simulink model "quad_drag_2015"  (Simulink 8.6)
settings: Solver=VariableStepAuto  StartTime=0.0  StopTime=100  RelTol=1e-3
settings Model: Creator=bsb  LastModifiedBy=bsb
settings DataIOCC: SaveFormat=Dataset  SignalLoggingSaveFormat=Dataset
settings OptimizationCC: ExpressionDepthLimit=128
settings DebuggingCC: UnderspecifiedInitializationDetection=Simplified  MergeDetectMultiDrivingBlocksExec=error  SolverPrmCheckMsg=none  FcnCallInpInsideContextMsg=EnableAllAsError  StateNameClashWarn=none
settings HardwareCC: ProdBitPerPointer=64  ProdLargestAtomicFloat=Float  ProdIntDivRoundTo=Zero  ProdEndianess=LittleEndian  ProdWordSize=64  ProdHWDeviceType=Intel->x86-64 (Windows64)
settings GRTTargetCC: GeneratePreprocessorConditionals=Use local settings  CombineOutputUpdateFcns=on  GRTInterface=off

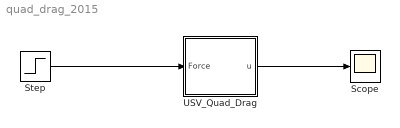
== system quad_drag_2015 ==
  Scope : Scope
  Step : Step  SampleTime=0
  USV_Quad_Drag : Subsystem
  wires:
  Step/1 -> USV_Quad_Drag/1(Force)
  USV_Quad_Drag/1(u) -> Scope/1

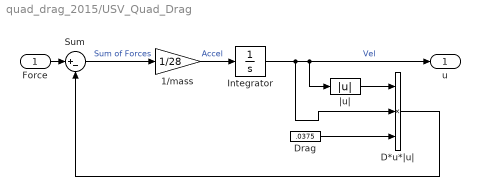
== system quad_drag_2015/USV_Quad_Drag ==
  Force : Inport
  1/mass : Gain  Gain=1/28
  D*u*|u| : Product  Inputs=3
  Drag : Constant  Value=.0375
  Integrator : Integrator
  Sum : Sum  Inputs=|+-
  |u| : Abs
  u : Outport
  wires:
  Integrator/1 -> D*u*|u|/2, u/1, |u|/1  "Vel"
  |u|/1 -> D*u*|u|/1
  Drag/1 -> D*u*|u|/3
  Force/1 -> Sum/1
  D*u*|u|/1 -> Sum/2
  Sum/1 -> 1/mass/1  "Sum of Forces"
  1/mass/1 -> Integrator/1  "Accel"
